simulink model "Channel"  (R2023b)
settings: Solver=VariableStepAuto  StartTime=0.0  StopTime=0.01  MaxStep=1e-3  RelTol=1e-3
libraries: simulink x6, dspsrcs4 x1, dspsigops x1
(part 3 of 3)

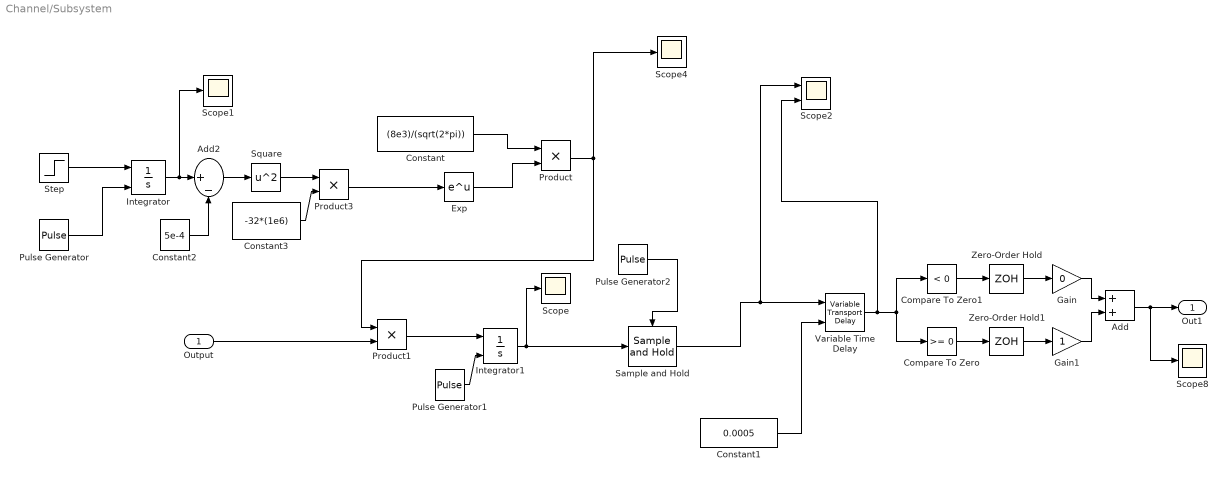
== system Channel/Subsystem ==
  Output : Inport
  Add : Sum
  Add2 : Sum  Inputs=|+-
  Compare To Zero : simulink/Logic and Bit Operations/Compare To Zero  relop=>=  OutDataTypeStr=boolean
  Compare To Zero1 : simulink/Logic and Bit Operations/Compare To Zero  relop=<  OutDataTypeStr=boolean
  Constant : Constant  Value=(8e3)/(sqrt(2*pi))  VectorParams1D=off
  Constant1 : Constant  Value=0.0005
  Constant2 : Constant  Value=5e-4
  Constant3 : Constant  Value=-32*(1e6)
  Exp : Math
  Gain : Gain  Gain=0
  Gain1 : Gain
  Integrator : Integrator  ExternalReset=rising
  Integrator1 : Integrator  ExternalReset=rising
  Product : Product
  Product1 : Product
  Product3 : Product
  Pulse Generator : DiscretePulseGenerator  PulseType=Time based  Period=1e-3  PulseWidth=5
  Pulse Generator1 : DiscretePulseGenerator  PulseType=Time based  Period=1e-3  PulseWidth=50
  Pulse Generator2 : DiscretePulseGenerator  PulseType=Time based  Period=1e-3  PulseWidth=50
  Sample and Hold : dspsigops/Sample and Hold  trig=Falling edge  initCond=0  latchinput=off
  Scope{,1,4,8} (4 alike) : Scope
  Scope2 : Scope  NumInputPorts=2
  Square : Math  Operator=square
  Step : Step  Time=0  SampleTime=0
  Variable Time Delay : VariableTransportDelay  MaximumDelay=0.5
  Zero-Order Hold : ZeroOrderHold  SampleTime=1e-3
  Zero-Order Hold1 : ZeroOrderHold  SampleTime=1e-3
  Out1 : Outport
  wires:
  Constant3/1 -> Product3/2
  Product3/1 -> Exp/1
  Square/1 -> Product3/1
  Integrator/1 -> Scope1/1, Add2/1
  Pulse Generator/1 -> Integrator/2
  Product/1 -> Product1/1, Scope4/1
  Constant2/1 -> Add2/2
  Step/1 -> Integrator/1
  Constant/1 -> Product/1
  Add2/1 -> Square/1
  Exp/1 -> Product/2
  Output/1 -> Product1/2
  Pulse Generator1/1 -> Integrator1/2
  Product1/1 -> Integrator1/1
  Integrator1/1 -> Scope/1, Sample and Hold/1
  Pulse Generator2/1 -> Sample and Hold/Trigger
  Compare To Zero/1 -> Zero-Order Hold1/1
  Constant1/1 -> Variable Time Delay/2
  Zero-Order Hold1/1 -> Gain1/1
  Variable Time Delay/1 -> Scope2/2, Compare To Zero1/1, Compare To Zero/1
  Zero-Order Hold/1 -> Gain/1
  Add/1 -> Out1/1, Scope8/1
  Gain/1 -> Add/1
  Gain1/1 -> Add/2
  Compare To Zero1/1 -> Zero-Order Hold/1
  Sample and Hold/1 -> Scope2/1, Variable Time Delay/1

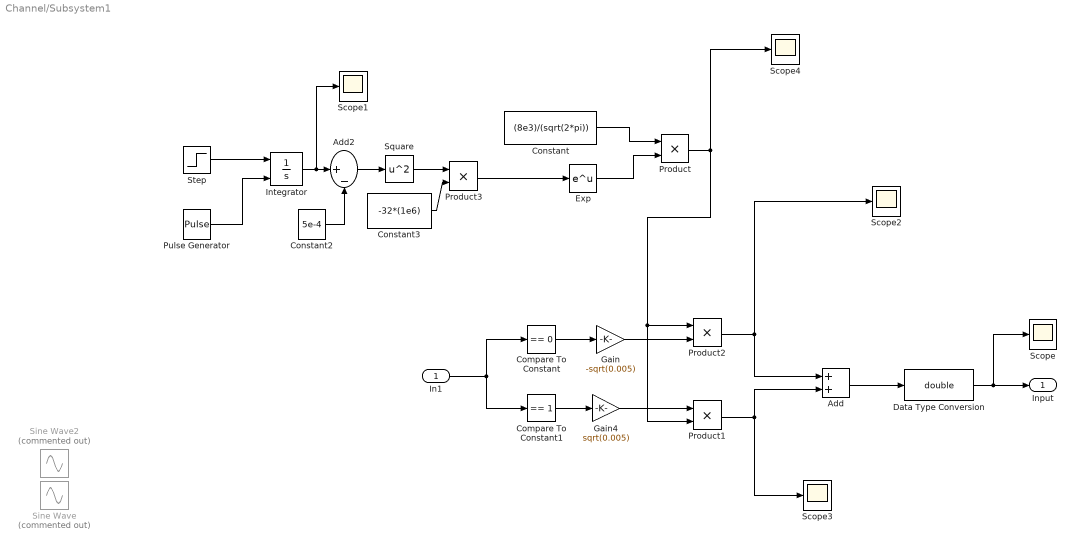
== system Channel/Subsystem1 ==
  In1 : Inport
  Add : Sum
  Add2 : Sum  Inputs=|+-
  Compare To Constant : simulink/Logic and Bit Operations/Compare To Constant  relop===  const=0  OutDataTypeStr=boolean
  Compare To Constant1 : simulink/Logic and Bit Operations/Compare To Constant  relop===  const=1  OutDataTypeStr=boolean
  Constant : Constant  Value=(8e3)/(sqrt(2*pi))  VectorParams1D=off
  Constant2 : Constant  Value=5e-4
  Constant3 : Constant  Value=-32*(1e6)
  Data Type Conversion : DataTypeConversion  OutDataTypeStr=double  SaturateOnIntegerOverflow=off  RndMeth=Floor  LockScale=on
  Exp : Math
  Gain : Gain  Gain=-sqrt(0.005)
  Gain4 : Gain  Gain=sqrt(0.005)
  Integrator : Integrator  ExternalReset=rising
  Product{,1..3} (4 alike) : Product
  Pulse Generator : DiscretePulseGenerator  PulseType=Time based  Period=1e-3  PulseWidth=5
  Scope{,1..4} (5 alike) : Scope
  Sine Wave : Sin  Commented=on  Amplitude=sqrt(2)  Frequency=1000*(2*pi)  Phase=pi/2  SampleTime=0.000001
  Sine Wave2 : Sin  Commented=on  Amplitude=sqrt(2)  Frequency=1000*(2*pi)  Phase=pi/2  SampleTime=0.000001
  Square : Math  Operator=square
  Step : Step  Time=0  SampleTime=0
  Input : Outport
  wires:
  Compare To Constant1/1 -> Gain4/1
  Constant2/1 -> Add2/2
  Square/1 -> Product3/1
  Constant/1 -> Product/1
  Exp/1 -> Product/2
  Constant3/1 -> Product3/2
  Product3/1 -> Exp/1
  Add2/1 -> Square/1
  Data Type Conversion/1 -> Scope/1, Input/1
  Add/1 -> Data Type Conversion/1
  In1/1 -> Compare To Constant1/1, Compare To Constant/1
  Compare To Constant/1 -> Gain/1
  Pulse Generator/1 -> Integrator/2
  Step/1 -> Integrator/1
  Integrator/1 -> Scope1/1, Add2/1
  Product/1 -> Product1/2, Product2/1, Scope4/1
  Product2/1 -> Scope2/1, Add/1
  Product1/1 -> Scope3/1, Add/2
  Gain/1 -> Product2/2
  Gain4/1 -> Product1/1

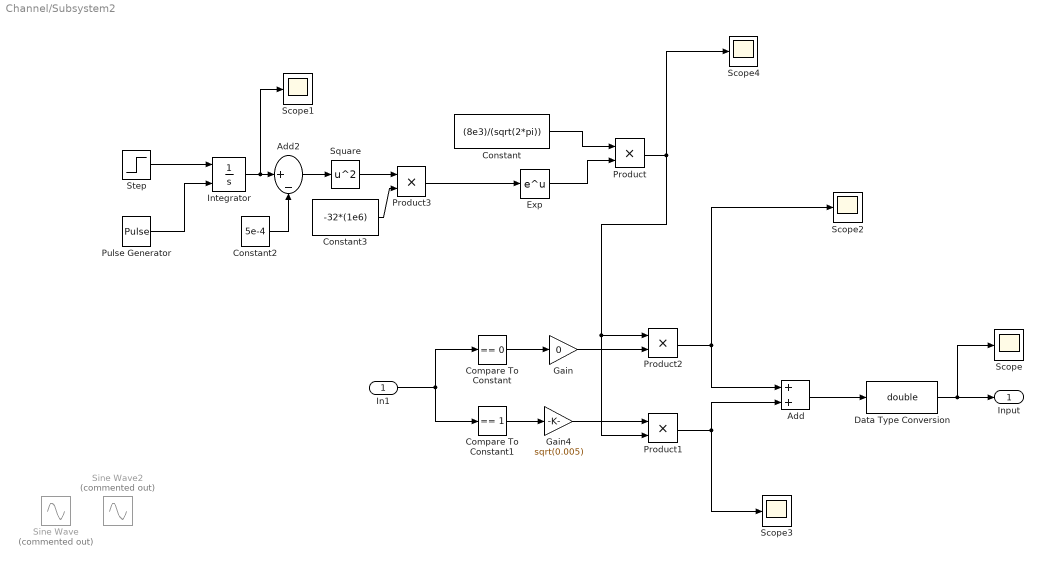
== system Channel/Subsystem2 ==
  In1 : Inport
  Add : Sum
  Add2 : Sum  Inputs=|+-
  Compare To Constant : simulink/Logic and Bit Operations/Compare To Constant  relop===  const=0  OutDataTypeStr=boolean
  Compare To Constant1 : simulink/Logic and Bit Operations/Compare To Constant  relop===  const=1  OutDataTypeStr=boolean
  Constant : Constant  Value=(8e3)/(sqrt(2*pi))  VectorParams1D=off
  Constant2 : Constant  Value=5e-4
  Constant3 : Constant  Value=-32*(1e6)
  Data Type Conversion : DataTypeConversion  OutDataTypeStr=double  SaturateOnIntegerOverflow=off  RndMeth=Floor  LockScale=on
  Exp : Math
  Gain : Gain  Gain=0
  Gain4 : Gain  Gain=sqrt(0.005)
  Integrator : Integrator  ExternalReset=rising
  Product{,1..3} (4 alike) : Product
  Pulse Generator : DiscretePulseGenerator  PulseType=Time based  Period=1e-3  PulseWidth=5
  Scope{,1..4} (5 alike) : Scope
  Sine Wave : Sin  Commented=on  Amplitude=sqrt(2)  Frequency=1000*(2*pi)  Phase=pi/2  SampleTime=0.000001
  Sine Wave2 : Sin  Commented=on  Amplitude=sqrt(2)  Frequency=1000*(2*pi)  Phase=pi/2  SampleTime=0.000001
  Square : Math  Operator=square
  Step : Step  Time=0  SampleTime=0
  Input : Outport
  wires:
  Compare To Constant1/1 -> Gain4/1
  Constant2/1 -> Add2/2
  Square/1 -> Product3/1
  Constant/1 -> Product/1
  Exp/1 -> Product/2
  Constant3/1 -> Product3/2
  Product3/1 -> Exp/1
  Add2/1 -> Square/1
  Data Type Conversion/1 -> Scope/1, Input/1
  Add/1 -> Data Type Conversion/1
  In1/1 -> Compare To Constant1/1, Compare To Constant/1
  Compare To Constant/1 -> Gain/1
  Pulse Generator/1 -> Integrator/2
  Step/1 -> Integrator/1
  Integrator/1 -> Scope1/1, Add2/1
  Product/1 -> Product1/2, Product2/1, Scope4/1
  Product2/1 -> Scope2/1, Add/1
  Product1/1 -> Scope3/1, Add/2
  Gain/1 -> Product2/2
  Gain4/1 -> Product1/1
